simulink model "PlantaSavePointPneuLongitudinalComCalculoVT"  (R2024b)
settings: Solver=ode23tb  StartTime=0.0  StopTime=100  MaxStep=0.01  RelTol=2e-3
values from neighbouring files (symbols this model uses):
  C1 = 1.2801    [CodigoSavePoint.m]    (also in CodigoVT.m)
  C2 = 23.99    [CodigoSavePoint.m]    (also in CodigoVT.m)
  C3 = 0.52    [CodigoSavePoint.m]    (also in CodigoVT.m)
undefined symbols (not defined in the file or in its folder): EV, MTR
libraries: autolibshared x5, slpidlib x2, autolibmappedmotor x2, vrlib x1, vehdynlibviscommon x1, vehdynlibscenariocommon x1, vehdynlibsteering x1, vehdynlibdriver x1
(part 4 of 4)

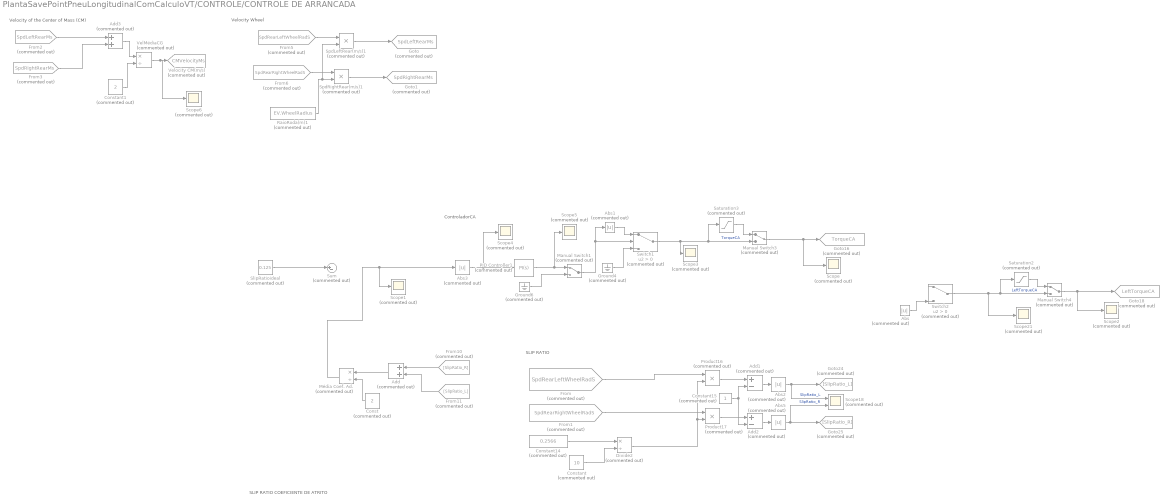
== system PlantaSavePointPneuLongitudinalComCalculoVT/CONTROLE/CONTROLE DE ARRANCADA  ==
  note: ControladorCA
  note: SLIP RATIO
  note: SLIP RATIO
      |
      | COEFICIENTE DE ATRITO
  note: Velocity of the Center of Mass (CM)
  note: Velocity Wheel
  Abs{,1..3,5} (5 alike) : Abs  Commented=on  SaturateOnIntegerOverflow=off
  Add : Sum  Commented=on
  Add1 : Sum  Commented=on  Inputs=+-
  Add2 : Sum  Commented=on  Inputs=+-
  Add3 : Sum  Commented=on
  Const : Constant  Commented=on  Value=2
  Constant : Constant  Commented=on  Value=10
  Constant1 : Constant  Commented=on  Value=2
  Constant14 : Constant  Commented=on  Value=0.2566  VectorParams1D=off
  Constant15 : Constant  Commented=on
  Divide2 : Product  Commented=on  Inputs=*/
  From : From  Commented=on  GotoTag=SpdRearLeftWheelRadS  TagVisibility=global
  From1 : From  Commented=on  GotoTag=SpdRearRightWheelRadS  TagVisibility=global
  From10 : From  Commented=on  GotoTag=SlipRatio_R
  From11 : From  Commented=on  GotoTag=SlipRatio_L
  From2 : From  Commented=on  GotoTag=SpdLeftRearMs  TagVisibility=global
  From3 : From  Commented=on  GotoTag=SpdRightRearMs  TagVisibility=global
  From5 : From  Commented=on  GotoTag=SpdRearLeftWheelRadS  TagVisibility=global
  From6 : From  Commented=on  GotoTag=SpdRearRightWheelRadS  TagVisibility=global
  Goto : Goto  Commented=on  GotoTag=SpdLeftRearMs  TagVisibility=global
  Goto1 : Goto  Commented=on  GotoTag=SpdRightRearMs  TagVisibility=global
  Goto16 : Goto  Commented=on  GotoTag=TorqueCA  TagVisibility=global
  Goto18 : Goto  Commented=on  GotoTag=LeftTorqueCA  TagVisibility=global
  Goto24 : Goto  Commented=on  GotoTag=SlipRatio_L
  Goto25 : Goto  Commented=on  GotoTag=SlipRatio_R
  Ground4 : Ground  Commented=on
  Ground6 : Ground  Commented=on
  Manual Switch1 : ManualSwitch  Commented=on
  Manual Switch3 : ManualSwitch  Commented=on
  Manual Switch4 : ManualSwitch  Commented=on
  Média Coef. Ad. : Product  Commented=on  Inputs=*/
  PID Controller1 : slpidlib/PID Controller  Commented=on  Controller=PI  Form=Parallel  TimeDomain=Continuous-time  UseExternalTs=off  SampleTime=-1  IntegratorMethod=Forward Euler  FilterMethod=Forward Euler  ControllerParametersSource=internal  P=0.01  I=0.01  UseKiTs=off  D=-1.04450033164761  UseExternalDerivativeSource=off  N=21.9051072982779  UseFilter=on  TunerSelectOption=Transfer Function Based (PID Tuner App)  InitialConditionSource=internal  InitialConditionForIntegrator=0  InitialConditionForFilter=0  DifferentiatorICPrevScaledInput=0  ExternalReset=none  TrackingMode=off  Kt=1  LimitOutput=off  SatLimitsSource=internal  UpperSaturationLimit=inf  LowerSaturationLimit=-inf  LinearizeAsGain=on  AntiWindupMode=none  Kb=1  LimitIntegrator=off  UpperIntegratorSaturationLimit=inf  LowerIntegratorSaturationLimit=-inf  POutMin=[]  POutMax=[]  IOutMin=[]  IOutMax=[]  DOutMin=[]  DOutMax=[]  NOutMin=[]  NOutMax=[]  SumOutMin=[]  SumOutMax=[]  SaturationOutMin=[]  SaturationOutMax=[]  PParamMin=[]  PParamMax=[]  IParamMin=[]  IParamMax=[]  DParamMin=[]  DParamMax=[]  NParamMin=[]  NParamMax=[]  KbParamMin=[]  KbParamMax=[]  KtParamMin=[]  KtParamMax=[]  KbOutMin=[]  KbOutMax=[]  KtOutMin=[]  KtOutMax=[]  IntegratorOutMin=[]  IntegratorOutMax=[]  FilterOutMin=[]  FilterOutMax=[]  SumI1OutMin=[]  SumI1OutMax=[]  SumI2OutMin=[]  SumI2OutMax=[]  SumI3OutMin=[]  SumI3OutMax=[]  SumI4OutMin=[]  SumI4OutMax=[]  SumDOutMin=[]  SumDOutMax=[]  DifferentiatorOutMin=[]  DifferentiatorOutMax=[]  FilterDiffOutCoefMin=[]  FilterDiffOutCoefMax=[]  ReciprocalOutMin=[]  ReciprocalOutMax=[]  SumDenOutMin=[]  SumDenOutMax=[]  SumNumOutMin=[]  SumNumOutMax=[]  DivideOutMin=[]  DivideOutMax=[]  UdiffTsProdOutMin=[]  UdiffTsProdOutMax=[]  NTsProdOutMin=[]  NTsProdOutMax=[]  UintegralTsProdOutMin=[]  UintegralTsProdOutMax=[]  UngainTsProdOutMin=[]  UngainTsProdOutMax=[]  ClampingZeroOutDataTypeStr=Inherit: Inherit via back propagation  ClampingZeroOutMin=[]  ClampingZeroOutMax=[]  FilterDenConstantOutDataTypeStr=Inherit: Inherit via back propagation  FilterDenConstantOutMin=[]  FilterDenConstantOutMax=[]  PCopyOutDataTypeStr=Inherit: Inherit via back propagation  PCopyOutMin=[]  PCopyOutMax=[]  NCopyOutDataTypeStr=Inherit: Inherit via back propagation  NCopyOutMin=[]  NCopyOutMax=[]  IntegratorContinuousStateAttributes=''  IntegratorStateMustResolveToSignalObject=off  IntegratorRTWStateStorageClass=Auto  FilterContinuousStateAttributes=''  FilterStateMustResolveToSignalObject=off  FilterRTWStateStorageClass=Auto  ParallelPVariant=InternalParameters  IdealPVariant=Disabled  IVariant=InternalParameters  DVariant=Disabled  IntegratorVariant=Continuous  SatVariant=Disabled  AWVariant=Passthrough  PCopyVariant=Disabled  TRVariant=Disabled  FdbkBlocksVariant=Forward  IdealPFdbkVariant=Disabled  SatFdbkVariant=Disabled  DerivativeFilterVariant=Disabled  NVariant=Disabled  NCopyVariant=Disabled_SignalSpec  FilterICVariant=Disabled  IntegratorICVariant=InternalICs  ExternalResetVariant=Disabled  TRSumVariant=Passthrough  SumFdbkVariant=Disabled  SumVariant=Sum_PI  TsampFilterVariant=InternalTs  TsampNgainVariant=Passthrough  TsampIntegralVariant=Disabled_SignalSpec  ExternalSaturationOutDataTypeStr=Inherit: Same as second input  DerivativeSourceVariant=Disabled  PreIntVariant=InternalPreInt
  Product16 : Product  Commented=on
  Product17 : Product  Commented=on
  RaioRoda(m)1 : Constant  Commented=on  Value=EV.WheelRadius  VectorParams1D=off
  Saturation2 : Saturate  Commented=on  UpperLimit=11.7  LowerLimit=0
  Saturation3 : Saturate  Commented=on  UpperLimit=11.7  LowerLimit=0
  Scope{,1..6,21} (8 alike) : Scope  Commented=on
  Scope18 : Scope  Commented=on  NumInputPorts=2
  SlipRatioideal : Constant  Commented=on  Value=0.125
  SpdLeftRear(m/s)1 : Product  Commented=on
  SpdRightRear(m/s)1 : Product  Commented=on
  Sum : Sum  Commented=on  Inputs=|+-
  Switch1 : Switch  Commented=on  Criteria=u2 > Threshold  SaturateOnIntegerOverflow=off  InputSameDT=off
  Switch2 : Switch  Commented=on  Criteria=u2 > Threshold  SaturateOnIntegerOverflow=off  InputSameDT=off
  VelMédiaCG : Product  Commented=on  Inputs=*/
  Velocity CM(m/s) : Goto  Commented=on  GotoTag=CMVelocityMs  TagVisibility=global
  wires:
  Add1/1 -> Abs2/1
  Divide2/1 -> Product16/2, Product17/2
  Manual Switch4/1 -> Scope2/1, Goto18/1
  SlipRatioideal/1 -> Sum/1
  Abs1/1 -> Switch1/1
  From11/1 -> Add/2
  From1/1 -> Product17/1
  Add/1 -> Média Coef. Ad./1
  Saturation3/1 -> Manual Switch3/1
  Constant15/1 -> Add1/2, Add2/2
  Ground6/1 -> Manual Switch1/2
  Ground4/1 -> Switch1/3
  Abs3/1 -> Scope4/1, PID Controller1/1
  Const/1 -> Média Coef. Ad./2
  Switch2/1 -> Saturation2/1, Manual Switch4/2, Scope21/1  "LeftTorqueCA"
  Saturation2/1 -> Manual Switch4/1
  Product17/1 -> Add2/1
  PID Controller1/1 -> Scope5/1, Manual Switch1/1
  From/1 -> Product16/1
  Switch1/1 -> Scope3/1, Saturation3/1, Manual Switch3/2  "TorqueCA"
  Manual Switch3/1 -> Scope/1, Goto16/1
  Product16/1 -> Add1/1
  Manual Switch1/1 -> Abs1/1, Switch1/2
  From10/1 -> Add/1
  Abs5/1 -> Scope18/2, Goto25/1  "SlipRatio_R"
  Add2/1 -> Abs5/1
  Abs2/1 -> Scope18/1, Goto24/1  "SlipRatio_L"
  Abs/1 -> Switch2/3
  From3/1 -> Add3/2
  VelMédiaCG/1 -> Scope6/1, Velocity CM(m/s)/1
  Constant1/1 -> VelMédiaCG/2
  Add3/1 -> VelMédiaCG/1
  From2/1 -> Add3/1
  Constant14/1 -> Divide2/1
  Constant/1 -> Divide2/2
  SpdRightRear(m/s)1/1 -> Goto1/1
  RaioRoda(m)1/1 -> SpdLeftRear(m/s)1/2, SpdRightRear(m/s)1/2
  SpdLeftRear(m/s)1/1 -> Goto/1
  From5/1 -> SpdLeftRear(m/s)1/1
  From6/1 -> SpdRightRear(m/s)1/1
  Média Coef. Ad./1 -> Scope1/1, Abs3/1

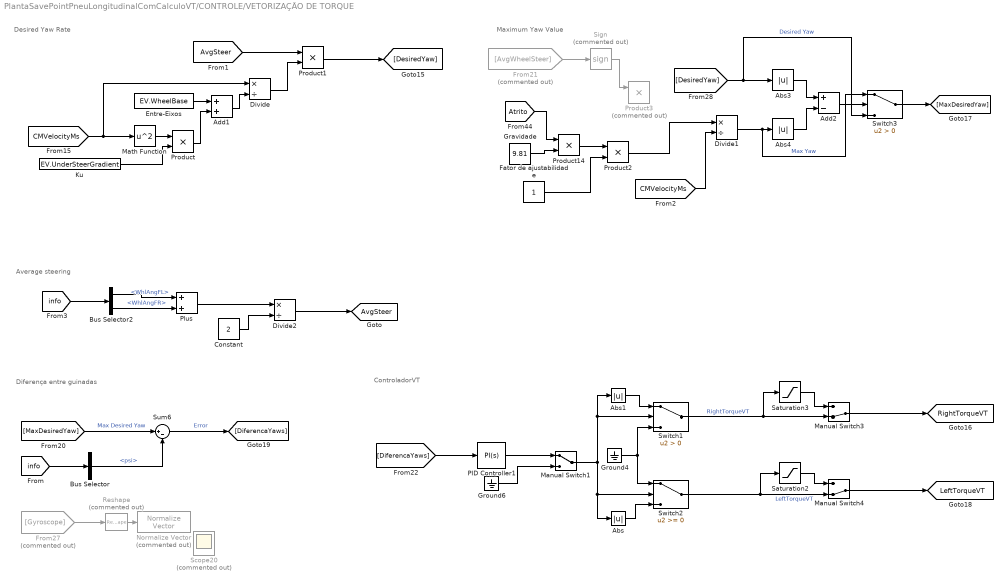
== system PlantaSavePointPneuLongitudinalComCalculoVT/CONTROLE/VETORIZAÇÃO DE TORQUE  ==
  note: ControladorVT
  note: Desired Yaw Rate
  note: Maximum Yaw Value
  note: Average steering
  note: Diferença entre guinadas
  Abs{,1,3..4} (4 alike) : Abs  SaturateOnIntegerOverflow=off
  Add1 : Sum
  Add2 : Sum  Inputs=+-
  Bus Selector : BusSelector  OutputSignals=InertFrm.Cg.Ang.psi
  Bus Selector2 : BusSelector  OutputSignals=BdyFrm.FrntAxl.Steer.WhlAngFL,BdyFrm.FrntAxl.Steer.WhlAngFR
  Constant : Constant  Value=2
  Divide : Product  Inputs=*/
  Divide1 : Product  Inputs=*/
  Divide2 : Product  Inputs=*/
  Entre-Eixos : Constant  Value=EV.WheelBase
  Fator de ajustabilidade : Constant
  From21 : From  Commented=on  GotoTag=AvgWheelSteer
  From27 : From  Commented=on  GotoTag=Gyroscope  TagVisibility=global
  Gravidade : Constant  Value=9.81
  Ground4 : Ground
  Ground6 : Ground
  Ku : Constant  Value=EV.UnderSteerGradient
  Manual Switch1 : ManualSwitch
  Manual Switch3 : ManualSwitch  CurrentSetting=0
  Manual Switch4 : ManualSwitch  CurrentSetting=0
  Math Function : Math  Operator=square
  Normalize Vector : vrlib/Utilities/Normalize Vector  Commented=on  maxzero=0
  PID Controller1 : slpidlib/PID Controller  Controller=PI  Form=Parallel  TimeDomain=Continuous-time  UseExternalTs=off  SampleTime=-1  IntegratorMethod=Forward Euler  FilterMethod=Forward Euler  ControllerParametersSource=internal  P=151.324360455076  I=15.2218532582345  UseKiTs=off  D=-1.04450033164761  UseExternalDerivativeSource=off  N=21.9051072982779  UseFilter=on  TunerSelectOption=Transfer Function Based (PID Tuner App)  InitialConditionSource=internal  InitialConditionForIntegrator=0  InitialConditionForFilter=0  DifferentiatorICPrevScaledInput=0  ExternalReset=none  TrackingMode=off  Kt=1  LimitOutput=off  SatLimitsSource=internal  UpperSaturationLimit=inf  LowerSaturationLimit=-inf  LinearizeAsGain=on  AntiWindupMode=none  Kb=1  LimitIntegrator=off  UpperIntegratorSaturationLimit=inf  LowerIntegratorSaturationLimit=-inf  POutMin=[]  POutMax=[]  IOutMin=[]  IOutMax=[]  DOutMin=[]  DOutMax=[]  NOutMin=[]  NOutMax=[]  SumOutMin=[]  SumOutMax=[]  SaturationOutMin=[]  SaturationOutMax=[]  PParamMin=[]  PParamMax=[]  IParamMin=[]  IParamMax=[]  DParamMin=[]  DParamMax=[]  NParamMin=[]  NParamMax=[]  KbParamMin=[]  KbParamMax=[]  KtParamMin=[]  KtParamMax=[]  KbOutMin=[]  KbOutMax=[]  KtOutMin=[]  KtOutMax=[]  IntegratorOutMin=[]  IntegratorOutMax=[]  FilterOutMin=[]  FilterOutMax=[]  SumI1OutMin=[]  SumI1OutMax=[]  SumI2OutMin=[]  SumI2OutMax=[]  SumI3OutMin=[]  SumI3OutMax=[]  SumI4OutMin=[]  SumI4OutMax=[]  SumDOutMin=[]  SumDOutMax=[]  DifferentiatorOutMin=[]  DifferentiatorOutMax=[]  FilterDiffOutCoefMin=[]  FilterDiffOutCoefMax=[]  ReciprocalOutMin=[]  ReciprocalOutMax=[]  SumDenOutMin=[]  SumDenOutMax=[]  SumNumOutMin=[]  SumNumOutMax=[]  DivideOutMin=[]  DivideOutMax=[]  UdiffTsProdOutMin=[]  UdiffTsProdOutMax=[]  NTsProdOutMin=[]  NTsProdOutMax=[]  UintegralTsProdOutMin=[]  UintegralTsProdOutMax=[]  UngainTsProdOutMin=[]  UngainTsProdOutMax=[]  ClampingZeroOutDataTypeStr=Inherit: Inherit via back propagation  ClampingZeroOutMin=[]  ClampingZeroOutMax=[]  FilterDenConstantOutDataTypeStr=Inherit: Inherit via back propagation  FilterDenConstantOutMin=[]  FilterDenConstantOutMax=[]  PCopyOutDataTypeStr=Inherit: Inherit via back propagation  PCopyOutMin=[]  PCopyOutMax=[]  NCopyOutDataTypeStr=Inherit: Inherit via back propagation  NCopyOutMin=[]  NCopyOutMax=[]  IntegratorContinuousStateAttributes=''  IntegratorStateMustResolveToSignalObject=off  IntegratorRTWStateStorageClass=Auto  FilterContinuousStateAttributes=''  FilterStateMustResolveToSignalObject=off  FilterRTWStateStorageClass=Auto  ParallelPVariant=InternalParameters  IdealPVariant=Disabled  IVariant=InternalParameters  DVariant=Disabled  IntegratorVariant=Continuous  SatVariant=Disabled  AWVariant=Passthrough  PCopyVariant=Disabled  TRVariant=Disabled  FdbkBlocksVariant=Forward  IdealPFdbkVariant=Disabled  SatFdbkVariant=Disabled  DerivativeFilterVariant=Disabled  NVariant=Disabled  NCopyVariant=Disabled_SignalSpec  FilterICVariant=Disabled  IntegratorICVariant=InternalICs  ExternalResetVariant=Disabled  TRSumVariant=Passthrough  SumFdbkVariant=Disabled  SumVariant=Sum_PI  TsampFilterVariant=InternalTs  TsampNgainVariant=Passthrough  TsampIntegralVariant=Disabled_SignalSpec  ExternalSaturationOutDataTypeStr=Inherit: Same as second input  DerivativeSourceVariant=Disabled  PreIntVariant=InternalPreInt
  Plus : Sum
  Product{,1..2,14} (4 alike) : Product
  Product3 : Product  Commented=on
  Reshape : Reshape  Commented=on
  Saturation2 : Saturate  UpperLimit=11.7  LowerLimit=0
  Saturation3 : Saturate  UpperLimit=11.7  LowerLimit=0
  Scope20 : Scope  Commented=on
  Sign : Signum  Commented=on
  Sum6 : Sum  Inputs=|+-
  Switch1 : Switch  Criteria=u2 > Threshold  SaturateOnIntegerOverflow=off  InputSameDT=off
  Switch2 : Switch  SaturateOnIntegerOverflow=off  InputSameDT=off
  Switch3 : Switch  Criteria=u2 > Threshold  SaturateOnIntegerOverflow=off  InputSameDT=off
  tag scope: AvgSteer=global, LeftTorqueVT=global, RightTorqueVT=global
  wires:
  Manual Switch3/1 -> [RightTorqueVT]
  Abs/1 -> Switch2/3
  Ground4/1 -> Switch1/3, Switch2/1
  PID Controller1/1 -> Manual Switch1/1
  Saturation3/1 -> Manual Switch3/1
  Switch1/1 -> Saturation3/1, Manual Switch3/2  "RightTorqueVT"
  Abs1/1 -> Switch1/1
  Manual Switch1/1 -> Abs/1, Switch2/2, Abs1/1, Switch1/2
  Ground6/1 -> Manual Switch1/2
  Manual Switch4/1 -> [LeftTorqueVT]
  Switch2/1 -> Saturation2/1, Manual Switch4/2  "LeftTorqueVT"
  Saturation2/1 -> Manual Switch4/1
  [DiferencaYaws] -> PID Controller1/1
  Product/1 -> Add1/2
  [AvgSteer] -> Product1/1
  Ku/1 -> Product/2
  Product1/1 -> [DesiredYaw]
  Math Function/1 -> Product/1
  [CMVelocityMs] -> Divide/1, Math Function/1
  Divide/1 -> Product1/2
  Entre-Eixos/1 -> Add1/1
  Add1/1 -> Divide/2
  From21/1 -> Sign/1
  Divide1/1 -> Switch3/1, Abs4/1  "Max Yaw"
  Switch3/1 -> [MaxDesiredYaw]
  [DesiredYaw] -> Abs3/1, Switch3/3  "Desired Yaw"
  Product2/1 -> Divide1/1
  Fator de ajustabilidade/1 -> Product2/2
  [CMVelocityMs] -> Divide1/2
  [Atrito] -> Product14/1
  Abs4/1 -> Add2/2
  Product14/1 -> Product2/1
  Sign/1 -> Product3/1
  Gravidade/1 -> Product14/2
  Abs3/1 -> Add2/1
  Add2/1 -> Switch3/2
  Bus Selector2/2 -> Plus/2  "<WhlAngFR>"
  Bus Selector2/1 -> Plus/1  "<WhlAngFL>"
  Constant/1 -> Divide2/2
  Divide2/1 -> [AvgSteer]
  Plus/1 -> Divide2/1
  [info] -> Bus Selector2/1
  Reshape/1 -> Normalize Vector/1
  Sum6/1 -> [DiferencaYaws]  "Error"
  [info] -> Bus Selector/1
  Bus Selector/1 -> Sum6/2  "<psi>"
  [MaxDesiredYaw] -> Sum6/1  "Max Desired Yaw"
  From27/1 -> Reshape/1

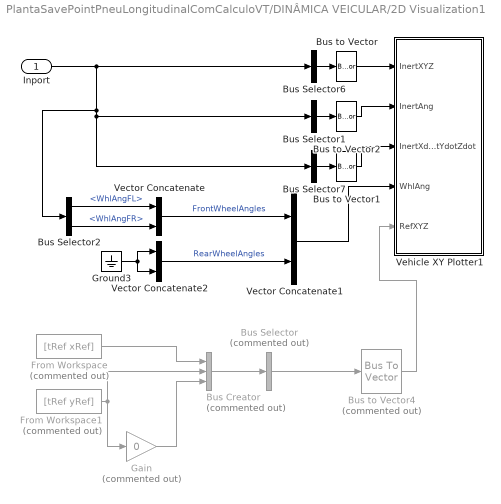
== system PlantaSavePointPneuLongitudinalComCalculoVT/DINÂMICA VEICULAR/2D Visualization1 ==
  Inport : Inport
  Bus Creator : BusCreator  Commented=on  Inputs=3
  Bus Selector : BusSelector  Commented=on  OutputSignals=signal1,signal2,signal3  OutputAsBus=on
  Bus Selector1 : BusSelector  OutputSignals=InertFrm.Cg.Ang.phi,InertFrm.Cg.Ang.theta,InertFrm.Cg.Ang.psi  OutputAsBus=on
  Bus Selector2 : BusSelector  OutputSignals=BdyFrm.FrntAxl.Steer.WhlAngFL,BdyFrm.FrntAxl.Steer.WhlAngFR
  Bus Selector6 : BusSelector  OutputSignals=InertFrm.Geom.Disp.X,InertFrm.Geom.Disp.Y,InertFrm.Geom.Disp.Z  OutputAsBus=on
  Bus Selector7 : BusSelector  OutputSignals=InertFrm.Geom.Vel.Xdot,InertFrm.Geom.Vel.Ydot,InertFrm.Geom.Vel.Zdot  OutputAsBus=on
  Bus to Vector : BusToVector
  Bus to Vector1 : BusToVector
  Bus to Vector2 : BusToVector
  Bus to Vector4 : BusToVector  Commented=on
  From Workspace : FromWorkspace  Commented=on  VariableName=[tRef xRef]
  From Workspace1 : FromWorkspace  Commented=on  VariableName=[tRef yRef]
  Gain : Gain  Commented=on  Gain=0
  Ground3 : Ground
  Vector Concatenate : Concatenate
  Vector Concatenate1 : Concatenate
  Vector Concatenate2 : Concatenate
  Vehicle XY Plotter1 : Subsystem  mask(Vehicle XY Plotter){extRef=on, extStats=off, extTireF=off, a=EV.FrontAxlePositionfromCG, b=EV.RearAxlePositionfromCG, w=2, figBorder=10, bufferSize=1024, velNorm=5, tireFNorm=1000, pltDT=0.2}
      mask prompts: extRef "Plot path reference, extRef"; extStats "Display speed, RPM and Gear"; extTireF "Display tire forces"; a "Distance to front axle from CG, a [m]:"; b "Distance to rear axle from CG, b [m]:"; w "Track width, w [m]:"; figBorder "Distance to figure borders, figBorder [m]:"; bufferSize "Path buffer sampe size, bufferSize []:"; velNorm "Velocity vector scaling, velNorm [m*s/m]:"; tireFNorm "Tire force vector scaling, tireFNorm [m/N]:"; pltDT "Plot update rate, pltDT [s]:"
      mask help:
      | This block will display a MATLAB figure which indicates the vehicle path, current position and heading velocity.
      | An optional path reference is also provided.
      mask init:
      | block = gcb;
      | if autoblkschecksimstopped(block)
      |     ParamNames = {'extRef';'extStats';'extTireF';'extTireF'};
      |     PortNames = {'RefXYZ';'Stats';'TireFx';'TireFy'};
      |     for idx=1:length(PortNames)
      |         InportOption  = {'built-in/Ground', [PortNames{idx}, ' Ground'];...
      |             'built-in/Inport',PortNames{idx}};
      |         if ~strcmp(get_param(block,ParamNames{idx}),'on')
      |             NewBlkHdl = autoblksreplaceblock(block, InportOption, 1);
      |             set_param(NewBlkHdl, 'ShowName', 'off');
      |         else
      |             autoblksreplaceblock(block, InportOption, 2);
      |         end
      |     end
      |     InportNames = {'InertXYZ';'InertAng';'InertXdotYdotZdot';'WhlAng';'RefXYZ';'Stats';'TireFx';'TireFy'};
      |     FoundNames = get_param(find_system(block, 'LookUnderMasks', 'all', 'SearchDepth', 1, 'FollowLinks', 'on', 'BlockType', 'Inport'), 'Name');
      |     [~,PortI] = intersect(InportNames, FoundNames);
      |     PortI = sort(PortI);
      |     for idx = 1:length(PortI)
      |         set_param([block, '/', InportNames{PortI(idx)}], 'Port', num2str(idx));
      |     end
      | end
      mask TypeOptions a: Vehicle XY Plotter/a
      mask TypeOptions b: Vehicle XY Plotter/b
      mask TypeOptions w: Vehicle XY Plotter/w
      mask TypeOptions figBorder: Vehicle XY Plotter/figBorder
      mask TypeOptions bufferSize: Vehicle XY Plotter/bufferSize
      mask TypeOptions velNorm: Vehicle XY Plotter/velNorm
      mask TypeOptions tireFNorm: Vehicle XY Plotter/tireFNorm
      mask DialogControl Container3 Prompt: Plot and Display Options
  wires:
  Vector Concatenate1/1 -> Vehicle XY Plotter1/4(WhlAng)
  Ground3/1 -> Vector Concatenate2/1, Vector Concatenate2/2
  Bus Selector6/1 -> Bus to Vector/1
  Vector Concatenate/1 -> Vector Concatenate1/1  "FrontWheelAngles"
  Vector Concatenate2/1 -> Vector Concatenate1/2  "RearWheelAngles"
  Bus Selector7/1 -> Bus to Vector1/1
  Bus to Vector1/1 -> Vehicle XY Plotter1/3(InertXdotYdotZdot)
  Bus to Vector/1 -> Vehicle XY Plotter1/1(InertXYZ)
  Bus to Vector2/1 -> Vehicle XY Plotter1/2(InertAng)
  Bus Selector1/1 -> Bus to Vector2/1
  Inport/1 -> Bus Selector2/1, Bus Selector7/1, Bus Selector1/1, Bus Selector6/1
  Bus to Vector4/1 -> Vehicle XY Plotter1/5(RefXYZ)
  Bus Selector/1 -> Bus to Vector4/1
  From Workspace1/1 -> Gain/1, Bus Creator/2
  Gain/1 -> Bus Creator/3
  From Workspace/1 -> Bus Creator/1
  Bus Creator/1 -> Bus Selector/1
  Bus Selector2/1 -> Vector Concatenate/1  "<WhlAngFL>"
  Bus Selector2/2 -> Vector Concatenate/2  "<WhlAngFR>"

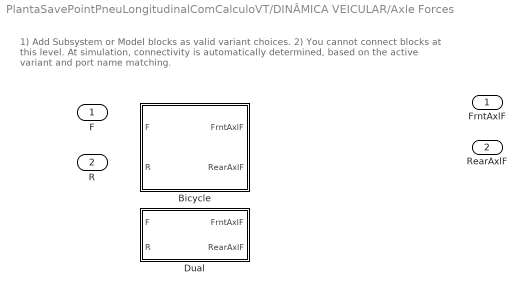
== system PlantaSavePointPneuLongitudinalComCalculoVT/DINÂMICA VEICULAR/Axle Forces ==
  note: 1) Add Subsystem or Model blocks as valid variant choices.
      | 2) You cannot connect blocks at this level. At simulation, connectivity is automatically
      | determined, based on the active variant and port name matching.
  F : Inport
  R : Inport  Port=2
  Bicycle : Subsystem  VariantControl=0
  Dual : Subsystem  VariantControl=1
  FrntAxlF : Outport  Unit=N  VectorParamsAs1DForOutWhenUnconnected=off
  RearAxlF : Outport  Port=2  Unit=N  VectorParamsAs1DForOutWhenUnconnected=off

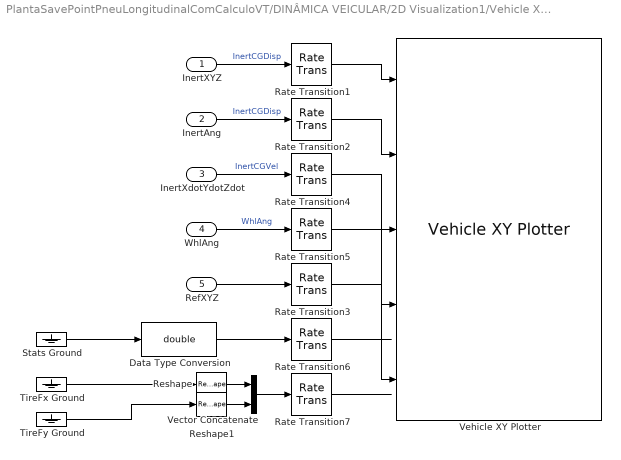
== system PlantaSavePointPneuLongitudinalComCalculoVT/DINÂMICA VEICULAR/2D Visualization1/Vehicle XY Plotter1 ==
  InertXYZ : Inport
  InertAng : Inport  Port=2
  InertXdotYdotZdot : Inport  Port=3
  WhlAng : Inport  Port=4
  RefXYZ : Inport  Port=5
  Data Type Conversion : DataTypeConversion  OutDataTypeStr=double  SaturateOnIntegerOverflow=off  RndMeth=Floor
  Rate Transition{1..7} (7 alike) : RateTransition  Deterministic=off  OutPortSampleTime=pltDT
  Reshape : Reshape  OutputDimensionality=Row vector (2-D)
  Reshape1 : Reshape  OutputDimensionality=Row vector (2-D)
  Stats Ground : Ground
  TireFx Ground : Ground
  TireFy Ground : Ground
  Vector Concatenate : Concatenate  Mode=Multidimensional array
  Vehicle XY Plotter : vehdynlibviscommon/Vehicle XY Plotter  w=w  a=a  b=b  figBorder=figBorder  bufferSize=bufferSize  extStats=off  extTireF=off
  wires:
  Vector Concatenate/1 -> Rate Transition7/1
  Reshape1/1 -> Vector Concatenate/2
  Reshape/1 -> Vector Concatenate/1
  RefXYZ/1 -> Rate Transition3/1
  Rate Transition7/1 -> ?
  Data Type Conversion/1 -> Rate Transition6/1
  Rate Transition6/1 -> ?
  Rate Transition5/1 -> Vehicle XY Plotter/4
  Rate Transition4/1 -> Vehicle XY Plotter/3
  Rate Transition2/1 -> Vehicle XY Plotter/2
  Rate Transition1/1 -> Vehicle XY Plotter/1
  Rate Transition3/1 -> Vehicle XY Plotter/5
  WhlAng/1 -> Rate Transition5/1  "WhlAng"
  InertXYZ/1 -> Rate Transition1/1  "InertCGDisp"
  InertXdotYdotZdot/1 -> Rate Transition4/1  "InertCGVel"
  InertAng/1 -> Rate Transition2/1  "InertCGDisp"
  Stats Ground/1 -> Data Type Conversion/1
  TireFx Ground/1 -> Reshape/1
  TireFy Ground/1 -> Reshape1/1

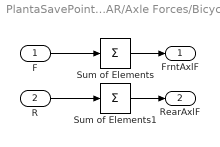
== system PlantaSavePointPneuLongitudinalComCalculoVT/DINÂMICA VEICULAR/Axle Forces/Bicycle ==
  F : Inport
  R : Inport  Port=2
  Sum of Elements : Sum  Inputs=+
  Sum of Elements1 : Sum  Inputs=+
  FrntAxlF : Outport  Unit=N  VectorParamsAs1DForOutWhenUnconnected=off
  RearAxlF : Outport  Port=2  Unit=N  VectorParamsAs1DForOutWhenUnconnected=off
  wires:
  Sum of Elements/1 -> FrntAxlF/1
  Sum of Elements1/1 -> RearAxlF/1
  R/1 -> Sum of Elements1/1
  F/1 -> Sum of Elements/1

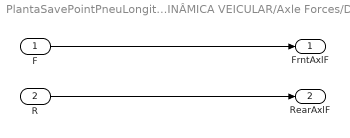
== system PlantaSavePointPneuLongitudinalComCalculoVT/DINÂMICA VEICULAR/Axle Forces/Dual ==
  F : Inport
  R : Inport  Port=2
  FrntAxlF : Outport  Unit=N  VectorParamsAs1DForOutWhenUnconnected=off
  RearAxlF : Outport  Port=2  Unit=N  VectorParamsAs1DForOutWhenUnconnected=off
  wires:
  R/1 -> RearAxlF/1
  F/1 -> FrntAxlF/1
